simulink model "simulation_2sim"  (R2022b)
settings: Solver=ode45  StartTime=0.0  StopTime=20  FixedStep=0.001  RelTol=1e-3  EnableMultiTasking=on
settings Model: Creator=Administrator  LastModifiedBy=Xheng
settings SolverCC: AlgebraicLoopSolver=TrustRegion
settings DataIOCC: SaveFormat=Array  SignalLoggingSaveFormat=ModelDataLogs  ReturnWorkspaceOutputs=off  SignalLoggingName=sigsOut
settings OptimizationCC: BooleanDataType=off  ExpressionDepthLimit=2147483647  InitFltsAndDblsToZero=on  LifeSpan=inf
settings DebuggingCC: SaveWithParameterizedLinksMsg=none  UnderspecifiedInitializationDetection=Classic  MergeDetectMultiDrivingBlocksExec=none  SignalResolutionControl=TryResolveAllWithWarning  MultiTaskDSMMsg=warning  MultiTaskCondExecSysMsg=none  FcnCallInpInsideContextMsg=warning  UnconnectedInputMsg=warning  UnconnectedOutputMsg=warning  UnconnectedLineMsg=warning  StateNameClashWarn=warning  SFUnexpectedBacktrackingDiag=warning  SFNoUnconditionalDefaultTransitionDiag=warning  SFExecutionAtInitializationDiag=none  SFMachineParentedDataDiag=warning  ArithmeticOperatorsInVariantConditions=warning
settings HardwareCC: ProdBitPerPointer=32  ProdBitPerSizeT=32  ProdBitPerPtrDiffT=32  ProdLargestAtomicFloat=None  ProdIntDivRoundTo=Undefined  ProdEndianess=Unspecified  ProdWordSize=32  ProdHWDeviceType=32-bit Generic  TargetUnknown=on
settings ModelReferenceCC: PropagateSignalLabelsOutOfModel=off
settings CodeAppCC: StateflowObjectComments=on
settings GRTTargetCC: TargetLangStandard=C89/C90 (ANSI)  CombineOutputUpdateFcns=off  GRTInterface=on
settings ConfigComp: CovMetricSettings=dw  CovSaveCumulativeToWorkspaceVar=on  CovSaveSingleToWorkspaceVar=on

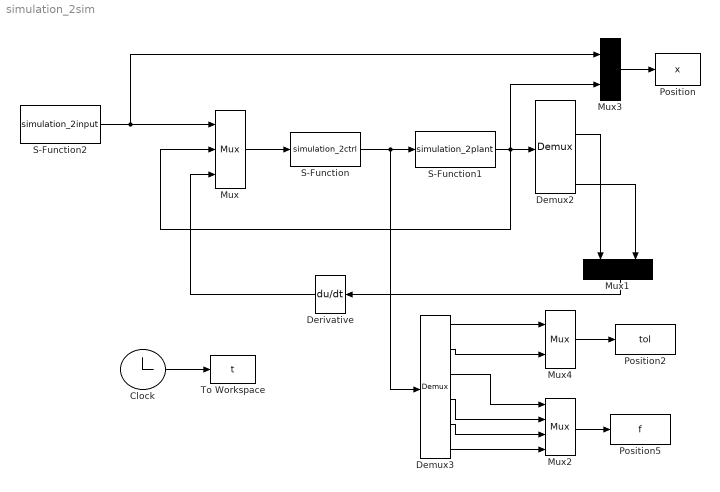
== system simulation_2sim ==
  Clock : Clock
  Demux2 : Demux
      settings: DisplayOption=none
  Demux3 : Demux  Outputs=6
      settings: DisplayOption=none
  Derivative : Derivative
  Mux : Mux  Inputs=3
  Mux1 : Mux  Inputs=2
  Mux2 : Mux
  Mux3 : Mux  Inputs=2
  Mux4 : Mux  Inputs=2
  Position : ToWorkspace  VariableName=x  SampleTime=-1
  Position2 : ToWorkspace  VariableName=tol  SampleTime=-1
  Position5 : ToWorkspace  VariableName=f  SampleTime=-1
  S-Function : S-Function  FunctionName=simulation_2ctrl  SFunctionDeploymentMode=off  EnableBusSupport=off
  S-Function1 : S-Function  FunctionName=simulation_2plant  SFunctionDeploymentMode=off  EnableBusSupport=off
  S-Function2 : S-Function  FunctionName=simulation_2input  SFunctionDeploymentMode=off  EnableBusSupport=off
  To Workspace : ToWorkspace  VariableName=t  SampleTime=-1
  wires:
  Mux/1 -> S-Function/1
  Mux3/1 -> Position/1
  S-Function/1 -> S-Function1/1, Demux3/1
  S-Function1/1 -> Demux2/1, Mux3/2, Mux/2
  S-Function2/1 -> Mux3/1, Mux/1
  Demux2/2 -> Mux1/1
  Demux2/4 -> Mux1/2
  Mux1/1 -> Derivative/1
  Derivative/1 -> Mux/3
  Clock/1 -> To Workspace/1
  Mux2/1 -> Position5/1
  Demux3/3 -> Mux2/1
  Demux3/4 -> Mux2/2
  Demux3/5 -> Mux2/3
  Demux3/6 -> Mux2/4
  Mux4/1 -> Position2/1
  Demux3/1 -> Mux4/1
  Demux3/2 -> Mux4/2
